simulink model "vid_vert_simulink"  (R2017b)
settings: Solver=FixedStepDiscrete  StartTime=0.0  StopTime=8  FixedStep=dt  RelTol=1e-3
values from neighbouring files (symbols this model uses):
  dt = [1 0.1 0.01 0.001]    [lab6.m]
undefined symbols (not defined in the file or in its folder): DiscIntNeverNeededParam, sig
settings Model: Creator=user  LastModifiedBy=user

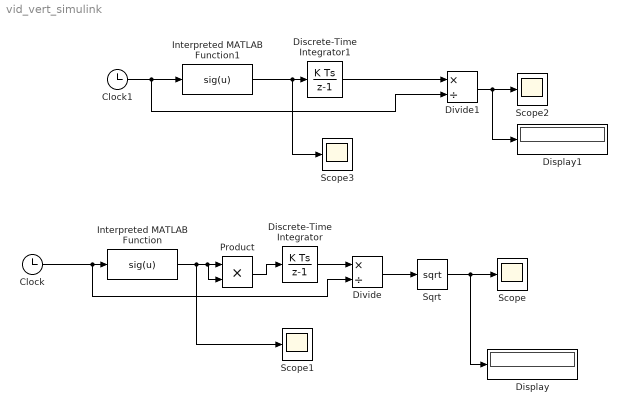
== system vid_vert_simulink ==
  Clock : Clock
  Clock1 : Clock
  Discrete-Time Integrator : DiscreteIntegrator  InitialConditionSetting=State (most efficient)  SampleTime=dt  ICPrevOutput=DiscIntNeverNeededParam  ICPrevScaledInput=DiscIntNeverNeededParam
  Discrete-Time Integrator1 : DiscreteIntegrator  InitialConditionSetting=State (most efficient)  SampleTime=dt  ICPrevOutput=DiscIntNeverNeededParam  ICPrevScaledInput=DiscIntNeverNeededParam
  Display : Display
  Display1 : Display
  Divide : Product  Inputs=*/
  Divide1 : Product  Inputs=*/
  Interpreted MATLAB Function : MATLABFcn  MATLABFcn=sig(u)
  Interpreted MATLAB Function1 : MATLABFcn  MATLABFcn=sig(u)
  Product : Product
  Scope{,1..3} (4 alike) : Scope
  Sqrt : Sqrt  SaturateOnIntegerOverflow=on
  wires:
  Clock/1 -> Divide/2, Interpreted MATLAB Function/1
  Interpreted MATLAB Function/1 -> Product/2, Product/1, Scope1/1
  Discrete-Time Integrator/1 -> Divide/1
  Divide/1 -> Sqrt/1
  Clock1/1 -> Divide1/2, Interpreted MATLAB Function1/1
  Interpreted MATLAB Function1/1 -> Scope3/1, Discrete-Time Integrator1/1
  Divide1/1 -> Display1/1, Scope2/1
  Sqrt/1 -> Scope/1, Display/1
  Product/1 -> Discrete-Time Integrator/1
  Discrete-Time Integrator1/1 -> Divide1/1
